simulink model "model_TugDynamics"  (R2023a)
settings: Solver=FixedStepAuto  StartTime=0.0  StopTime=400  FixedStep=0.025  RelTol=1e-3
model mask{StartTug=StartTug, Towline=0, Point=0}
  mask prompts: StartTug "Starting position [x y psi u v r]':"; Towline "Towline length:"; Point "Towline connection point Tanker [x_b y_b]':"
model workspace (MAT data in the model file):
  Point = [0; 0]
  Sig = Simulink.Signal
  Sig.DataType = 'auto'
  Sig.Dimensions = -1
  Sig.DimensionsMode = 'auto'
  Sig.Complexity = 'auto'
  Sig.SampleTime = -1
  Sig.SamplingMode = 'auto'
  StartTug = [0; 0; 0; 0; 0; 0]
  Towline = 0
  angleP = 0
  angleS = 0
  rpmP = 0
  rpmS = 0
undefined symbols (not defined in the file): TugStart
libraries: simulink x2
settings Model: ParameterArgumentNames=Point,StartTug,Towline  Creator=henni  LastModifiedBy=rkr021
settings OptimizationCC: ReuseModelBlockBuffer=off
settings DebuggingCC: UnconnectedInputMsg=warning  UnconnectedOutputMsg=warning  UnconnectedLineMsg=warning
settings ModelReferenceCC: EnableRefExpFcnMdlSchedulingChecks=on
settings RTWCC: DLArmComputeVersion=19.05

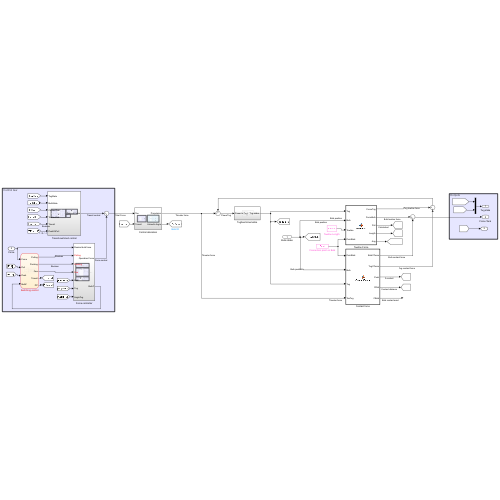
[thumbnail: Simulink's stored preview of the top-level diagram]
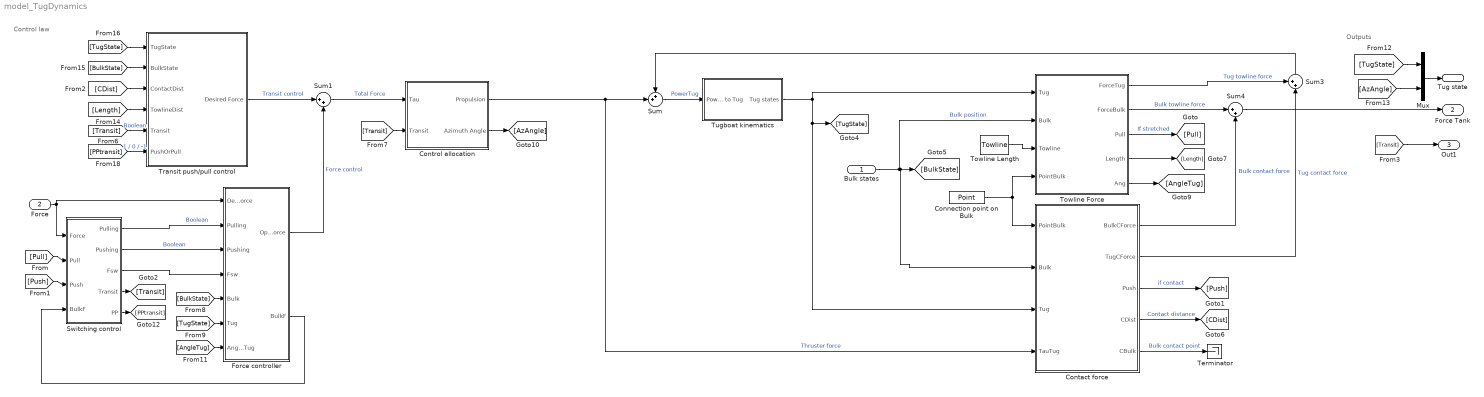
== system model_TugDynamics ==
  note: Outputs
  note: Control law
  Bulk states : Inport  PortDimensions=6
  Force : Inport  Port=2
  Connection point on Bulk : Constant  Value=Point
  Contact force : MATLAB Function  TreatAsAtomicUnit=on
  Control allocation : Subsystem
  Force controller : Subsystem
  Mux : Mux  Inputs=2
  Sum : Sum  Inputs=++|
  Sum1 : Sum  Inputs=|++
  Sum3 : Sum  Inputs=++|
  Sum4 : Sum  Inputs=|++
  Switching control : Stateflow chart  TreatAsAtomicUnit=on
  Terminator : Terminator
  Towline Force : MATLAB Function  TreatAsAtomicUnit=on
  Towline Length : Constant  Value=Towline
  Transit push/pull control : Subsystem
  Tugboat kinematics : Subsystem
  Tug state : Outport
  Force Tank : Outport  Port=2
  Out1 : Outport  Port=3
  wires:
  Sum3/1 -> Sum/1
  Tugboat kinematics/1(Tug states) -> Contact force/3(Tug), [TugState], Towline Force/1(Tug)
  Bulk states/1 -> [BulkState], Contact force/2(Bulk), Towline Force/2(Bulk)  "Bulk position"
  Sum4/1 -> Force Tank/1
  Towline Force/2(ForceBulk) -> Sum4/1  "Bulk towline force"
  Towline Length/1 -> Towline Force/3(Towline)
  Connection point on Bulk/1 -> Towline Force/4(PointBulk), Contact force/1(PointBulk)
  Contact force/1(BulkCForce) -> Sum4/2  "Bulk contact force"
  Towline Force/1(ForceTug) -> Sum3/1  "Tug towline force"
  Contact force/2(TugCForce) -> Sum3/2  "Tug contact force"
  Contact force/3(Push) -> [Push]  "if contact"
  Towline Force/3(Pull) -> [Pull]  "If stretched"
  Sum/1 -> Tugboat kinematics/1(Power to Tug)  "PowerTug"
  Control allocation/2(Azimuth Angle) -> [AzAngle]
  Control allocation/1(Propulsion) -> Contact force/4(TauTug), Sum/2  "Thruster force"
  Contact force/4(CDist) -> [CDist]  "Contact distance"
  Towline Force/4(Length) -> [Length]
  Contact force/5(CBulk) -> Terminator/1  "Bulk contact point"
  [Transit] -> Control allocation/2(Transit)
  Towline Force/5(Ang) -> [AngleTug]
  [TugState] -> Mux/1
  [AzAngle] -> Mux/2
  Mux/1 -> Tug state/1
  Switching control/3(Fsw) -> Force controller/4(Fsw)
  [PPtransit] -> Transit push/pull control/6(PushOrPull)  "1 / 0 / -1"
  [AngleTug] -> Force controller/7(AngleTug)
  [Push] -> Switching control/3(Push)
  [TugState] -> Force controller/6(Tug)
  Force/1 -> Switching control/1(Force), Force controller/1(Desired bulk force)
  Force controller/2(BulkF) -> Switching control/4(BulkF)
  Transit push/pull control/1(Desired Force) -> Sum1/1  "Transit control"
  [CDist] -> Transit push/pull control/3(ContactDist)
  [Transit] -> Transit push/pull control/5(Transit)  "Boolean"
  Switching control/2(Pushing) -> Force controller/3(Pushing)  "Boolean"
  [BulkState] -> Force controller/5(Bulk)
  Force controller/1(Operation Force) -> Sum1/2  "Force control"
  [Pull] -> Switching control/2(Pull)
  Switching control/5(PP) -> [PPtransit]
  Sum1/1 -> Control allocation/1(Tau)  "Total Force"
  Switching control/1(Pulling) -> Force controller/2(Pulling)  "Boolean"
  [Length] -> Transit push/pull control/4(TowlineDist)
  [TugState] -> Transit push/pull control/1(TugState)
  [BulkState] -> Transit push/pull control/2(BulkState)
  Switching control/4(Transit) -> [Transit]
  [Transit] -> Out1/1

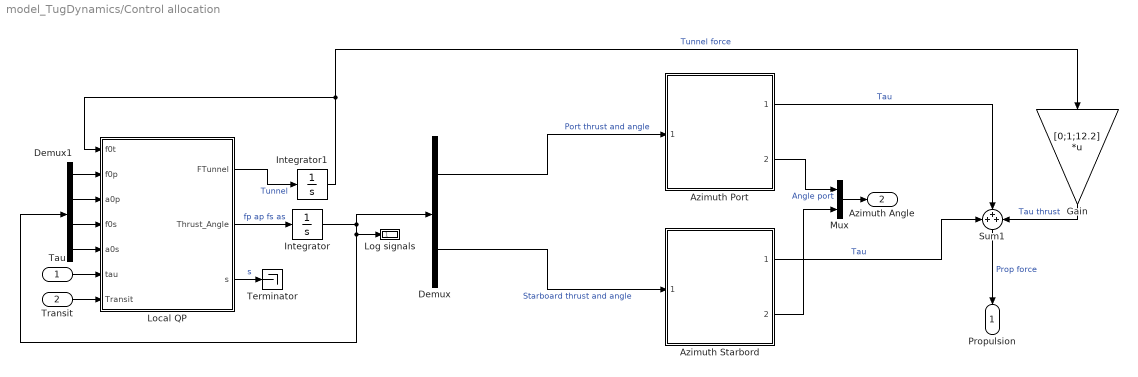
== system model_TugDynamics/Control allocation ==
  Tau : Inport  PortDimensions=3
  Transit : Inport  Port=2
  Azimuth Port : Subsystem  TreatAsAtomicUnit=on  ReferencedSubsystem=Subsystem_TugAzimuth  PosAz=[-13.9;-3]
  Azimuth Starbord : Subsystem  TreatAsAtomicUnit=on  ReferencedSubsystem=Subsystem_TugAzimuth  PosAz=[-13.9;3]
  Demux : Demux  Outputs=2
  Demux1 : Demux
  Gain : Gain  Gain=[0;1;12.2]  Multiplication=Matrix(K*u)
  Integrator : Integrator  InitialCondition=[0;deg2rad(0);0;deg2rad(-0)]
  Integrator1 : Integrator
  Local QP : MATLAB Function  TreatAsAtomicUnit=on
  Log signals : Subsystem
  Mux : Mux  Inputs=2
  Sum1 : Sum  Inputs=+++
  Terminator : Terminator
  Propulsion : Outport  PortDimensions=3
  Azimuth Angle : Outport  Port=2
  wires:
  Azimuth Port/1 -> Sum1/2  "Tau"
  Azimuth Starbord/1 -> Sum1/1  "Tau"
  Mux/1 -> Azimuth Angle/1
  Sum1/1 -> Propulsion/1  "Prop force"
  Demux/1 -> Azimuth Port/1  "Port thrust and angle"
  Integrator1/1 -> Gain/1, Local QP/1(f0t)  "Tunnel force"
  Integrator/1 -> Demux1/1, Log signals/1(Input), Demux/1
  Demux1/2 -> Local QP/3(a0p)
  Demux1/1 -> Local QP/2(f0p)
  Demux1/4 -> Local QP/5(a0s)
  Local QP/2(Thrust_Angle) -> Integrator/1  "fp ap fs as"
  Tau/1 -> Local QP/6(tau)
  Demux1/3 -> Local QP/4(f0s)
  Local QP/1(FTunnel) -> Integrator1/1  "Tunnel"
  Demux/2 -> Azimuth Starbord/1  "Starboard thrust and angle"
  Azimuth Port/2 -> Mux/1  "Angle port"
  Azimuth Starbord/2 -> Mux/2
  Transit/1 -> Local QP/7(Transit)
  Gain/1 -> Sum1/3  "Tau thrust"
  Local QP/3(s) -> Terminator/1  "s"

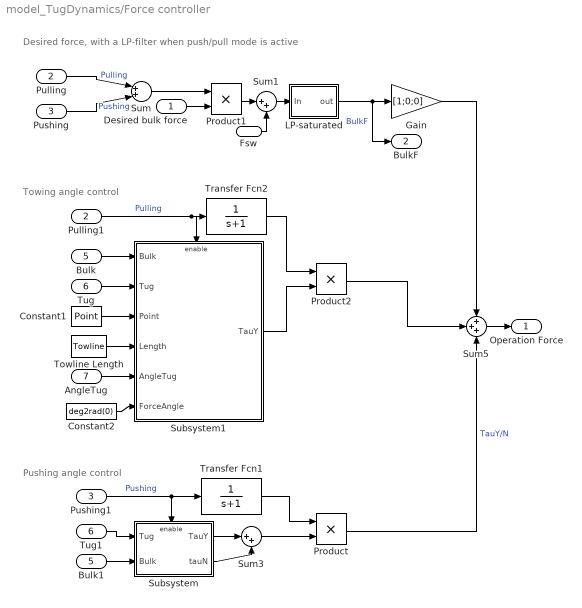
== system model_TugDynamics/Force controller ==
  note: Towing angle control
  note: Desired force, with a LP-filter when push/pull mode is active
  note: Pushing angle control
  Desired bulk force : Inport
  Pulling : Inport  Port=2
  Pushing : Inport  Port=3
  Fsw : Inport  Port=4
  Bulk : Inport  Port=5
  Tug : Inport  Port=6
  AngleTug : Inport  Port=7
  Bulk1 : InportShadow  Port=5
  Constant1 : Constant  Value=Point
  Constant2 : Constant  Value=deg2rad(0)
  Gain : Gain  Gain=[1;0;0]
  LP-saturated : Subsystem
  Product : Product
  Product1 : Product
  Product2 : Product
  Pulling1 : InportShadow  Port=2
  Pushing1 : InportShadow  Port=3
  Subsystem : Subsystem
  Subsystem1 : Subsystem
  Sum : Sum  Inputs=|++|
  Sum1 : Sum  Inputs=|++
  Sum3 : Sum  Inputs=|++
  Sum5 : Sum  Inputs=+++
  Towline Length : Constant  Value=Towline
  Transfer Fcn1 : TransferFcn  Denominator=[1 1]
  Transfer Fcn2 : TransferFcn  Denominator=[1 1]
  Tug1 : InportShadow  Port=6
  Operation Force : Outport
  BulkF : Outport  Port=2
  wires:
  Bulk1/1 -> Subsystem/2(Bulk)
  Pulling1/1 -> Subsystem1/Enable, Transfer Fcn2/1  "Pulling"
  Tug1/1 -> Subsystem/1(Tug)
  Constant1/1 -> Subsystem1/3(Point)
  Desired bulk force/1 -> Product1/2
  Transfer Fcn2/1 -> Product2/1
  Sum5/1 -> Operation Force/1
  Gain/1 -> Sum5/1
  Transfer Fcn1/1 -> Product/1
  Pulling/1 -> Sum/1  "Pulling"
  AngleTug/1 -> Subsystem1/5(AngleTug)
  Pushing/1 -> Sum/2  "Pushing"
  Bulk/1 -> Subsystem1/1(Bulk)
  Towline Length/1 -> Subsystem1/4(Length)
  Tug/1 -> Subsystem1/2(Tug)
  Product2/1 -> Sum5/2
  Product1/1 -> Sum1/1
  Fsw/1 -> Sum1/2
  LP-saturated/1(out) -> Gain/1, BulkF/1  "BulkF"
  Sum1/1 -> LP-saturated/1(In)
  Product/1 -> Sum5/3  "TauY/N"
  Constant2/1 -> Subsystem1/6(ForceAngle)
  Pushing1/1 -> Transfer Fcn1/1, Subsystem/Enable  "Pushing"
  Sum/1 -> Product1/1
  Subsystem/2(tauN) -> Sum3/2
  Subsystem/1(TauY) -> Sum3/1
  Sum3/1 -> Product/2
  Subsystem1/1(TauY) -> Product2/2

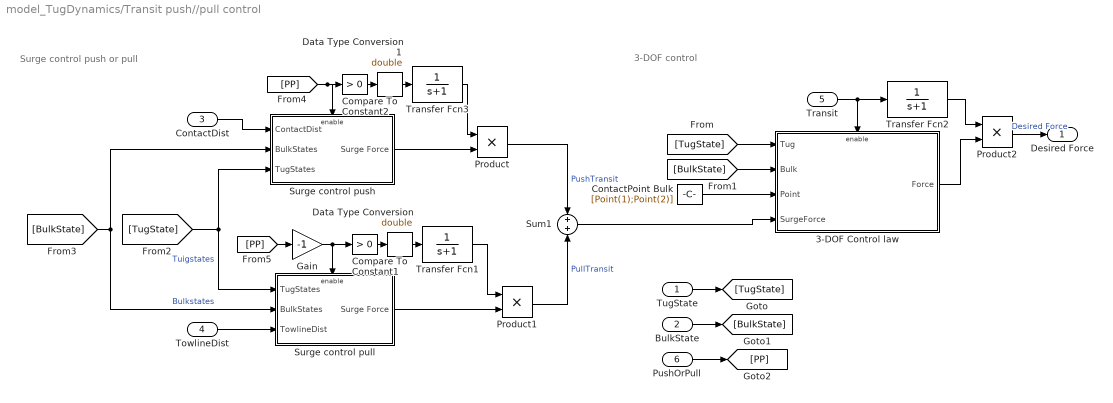
== system model_TugDynamics/Transit push//pull control ==
  note: 3-DOF control
  note: Surge control push or pull
  TugState : Inport
  BulkState : Inport  Port=2
  ContactDist : Inport  Port=3
  TowlineDist : Inport  Port=4
  Transit : Inport  Port=5
  PushOrPull : Inport  Port=6
  3-DOF Control law : Subsystem
  Compare To Constant1 : simulink/Logic and Bit Operations/Compare To Constant  relop=>  const=0  OutDataTypeStr=uint8
  Compare To Constant2 : simulink/Logic and Bit Operations/Compare To Constant  relop=>  const=0  OutDataTypeStr=uint8
  ContactPoint Bulk : Constant  Value=[Point(1);Point(2)]
  Data Type Conversion : DataTypeConversion  OutDataTypeStr=double  SaturateOnIntegerOverflow=off  RndMeth=Floor
  Data Type Conversion1 : DataTypeConversion  OutDataTypeStr=double  SaturateOnIntegerOverflow=off  RndMeth=Floor
  Gain : Gain  Gain=-1
  Product : Product
  Product1 : Product
  Product2 : Product
  Sum1 : Sum
  Surge control pull : Subsystem
  Surge control push : Subsystem
  Transfer Fcn1 : TransferFcn  Denominator=[1 1]
  Transfer Fcn2 : TransferFcn  Denominator=[1 1]
  Transfer Fcn3 : TransferFcn  Denominator=[1 1]
  Desired Force : Outport
  wires:
  [BulkState] -> Surge control pull/2(BulkStates), Surge control push/2(BulkStates)  "Bulkstates"
  Surge control pull/1(Surge Force) -> Product1/2
  [TugState] -> Surge control pull/1(TugStates), Surge control push/3(TugStates)  "Tuigstates"
  TowlineDist/1 -> Surge control pull/3(TowlineDist)
  ContactDist/1 -> Surge control push/1(ContactDist)
  TugState/1 -> [TugState]
  BulkState/1 -> [BulkState]
  PushOrPull/1 -> [PP]
  [PP] -> Compare To Constant2/1, Surge control push/Enable
  [PP] -> Gain/1
  Gain/1 -> Compare To Constant1/1, Surge control pull/Enable
  Surge control push/1(Surge Force) -> Product/2
  [TugState] -> 3-DOF Control law/1(Tug)
  [BulkState] -> 3-DOF Control law/2(Bulk)
  ContactPoint Bulk/1 -> 3-DOF Control law/3(Point)
  3-DOF Control law/1(" Force") -> Product2/2
  Transit/1 -> Transfer Fcn2/1, 3-DOF Control law/Enable
  Transfer Fcn3/1 -> Product/1
  Product/1 -> Sum1/1  "PushTransit"
  Compare To Constant1/1 -> Data Type Conversion/1
  Transfer Fcn1/1 -> Product1/1
  Product1/1 -> Sum1/2  "PullTransit"
  Transfer Fcn2/1 -> Product2/1
  Product2/1 -> Desired Force/1  "Desired Force"
  Sum1/1 -> 3-DOF Control law/4(SurgeForce)
  Data Type Conversion/1 -> Transfer Fcn1/1
  Data Type Conversion1/1 -> Transfer Fcn3/1
  Compare To Constant2/1 -> Data Type Conversion1/1

== system model_TugDynamics/Tugboat kinematics ==
  Power to Tug : Inport  PortDimensions=3
  Integrator : Integrator  InitialConditionSource=external  InitialCondition=[0;0;0;0;0;0]
  Kinematics CALC : MATLAB Function  TreatAsAtomicUnit=on
  initial state : Constant  Value=StartTug
  Tug states : Outport
  wires:
  Integrator/1 -> Kinematics CALC/1(x), Tug states/1  "x"
  Power to Tug/1 -> Kinematics CALC/2(tau)
  initial state/1 -> Integrator/2
  Kinematics CALC/1(xdot) -> Integrator/1  "xdot"

== system model_TugDynamics/Control allocation/Log signals ==
  Input : Inport
  Demux : Demux
  Gain1 : Gain  Gain=180/pi
  Gain2 : Gain  Gain=180/pi
  Mux1 : Mux
  Terminator : Terminator
  wires:
  Demux/2 -> Gain2/1  "Port angle"
  Mux1/1 -> Terminator/1  "PT PA ST SA"
  Gain2/1 -> Mux1/2  "Port angle"
  Demux/4 -> Gain1/1  "star angle"
  Gain1/1 -> Mux1/4  "star angle"
  Demux/3 -> Mux1/3  "Star thrust desired"
  Demux/1 -> Mux1/1  "Port Thrust desired"
  Input/1 -> Demux/1

== system model_TugDynamics/Force controller/LP-saturated ==
  In : Inport
  Integrator : Integrator
  Saturation : Saturate  UpperLimit=5e4  LowerLimit=-5e4
  Sum2 : Sum  Inputs=|+-
  out : Outport
  wires:
  Integrator/1 -> out/1, Sum2/2  "ut"
  Sum2/1 -> Saturation/1
  Saturation/1 -> Integrator/1
  In/1 -> Sum2/1

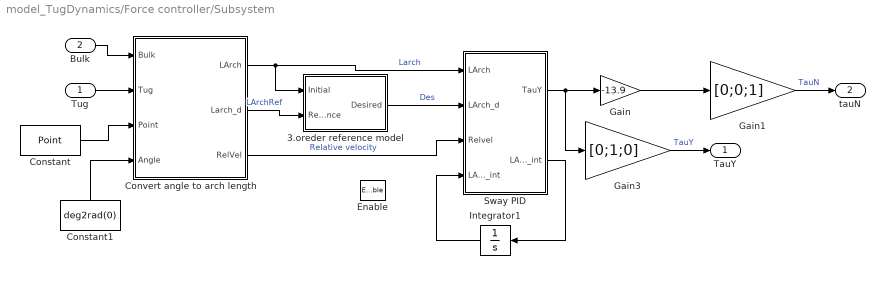
== system model_TugDynamics/Force controller/Subsystem ==
  Tug : Inport
  Bulk : Inport  Port=2
  Enable : EnablePort  StatesWhenEnabling=reset
  3.oreder reference model : Subsystem  mask{wn=0.02, zeta=1, sat_rd=0.4, sat_ad=0.01}
      mask prompts: wn "Natural frequency:"; zeta "Relative damping:"; sat_rd "Saturation eta_d_dot:"; sat_ad "Saturation eta_d_Ddot:"
  Constant : Constant  Value=Point
  Constant1 : Constant  Value=deg2rad(0)
  Convert angle to arch length : MATLAB Function  TreatAsAtomicUnit=on
  Gain : Gain  Gain=-13.9
  Gain1 : Gain  Gain=[0;0;1]
  Gain3 : Gain  Gain=[0;1;0]
  Integrator1 : Integrator
  Sway PID : MATLAB Function  TreatAsAtomicUnit=on
  TauY : Outport
  tauN : Outport  Port=2
  wires:
  Constant1/1 -> Convert angle to arch length/4(Angle)
  Gain1/1 -> tauN/1  "TauN"
  Gain3/1 -> TauY/1  "TauY"
  Tug/1 -> Convert angle to arch length/2(Tug)
  Constant/1 -> Convert angle to arch length/3(Point)
  Gain/1 -> Gain1/1
  Integrator1/1 -> Sway PID/4(LArch_int)
  Bulk/1 -> Convert angle to arch length/1(Bulk)
  Sway PID/2(LArch_error_int) -> Integrator1/1
  3.oreder reference model/1(Desired) -> Sway PID/2(LArch_d)  "Des"
  Convert angle to arch length/2(Larch_d) -> 3.oreder reference model/2(Reference)  "LArchRef"
  Convert angle to arch length/3(RelVel) -> Sway PID/3(Relvel)  "Relative velocity"
  Convert angle to arch length/1(LArch) -> 3.oreder reference model/1(Initial), Sway PID/1(LArch)  "Larch"
  Sway PID/1(TauY) -> Gain/1, Gain3/1

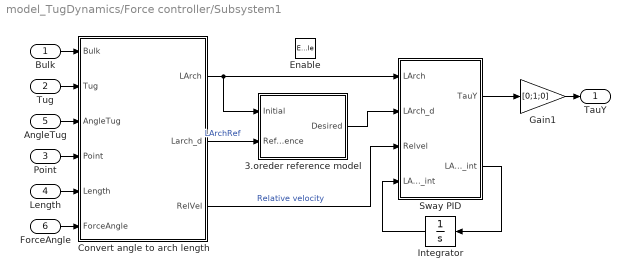
== system model_TugDynamics/Force controller/Subsystem1 ==
  Bulk : Inport
  Tug : Inport  Port=2
  Point : Inport  Port=3
  Length : Inport  Port=4
  AngleTug : Inport  Port=5
  ForceAngle : Inport  Port=6
  Enable : EnablePort  StatesWhenEnabling=reset
  3.oreder reference model : Subsystem  mask{wn=0.03, zeta=1, sat_rd=0.4, sat_ad=0.01}
      mask prompts: wn "Natural frequency:"; zeta "Relative damping:"; sat_rd "Saturation eta_d_dot:"; sat_ad "Saturation eta_d_Ddot:"
  Convert angle to arch length : MATLAB Function  TreatAsAtomicUnit=on
  Gain1 : Gain  Gain=[0;1;0]
  Integrator : Integrator
  Sway PID : MATLAB Function  TreatAsAtomicUnit=on
  TauY : Outport
  wires:
  Convert angle to arch length/1(LArch) -> Sway PID/1(LArch), 3.oreder reference model/1(Initial)
  Tug/1 -> Convert angle to arch length/2(Tug)
  ForceAngle/1 -> Convert angle to arch length/6(ForceAngle)
  Sway PID/1(TauY) -> Gain1/1
  Point/1 -> Convert angle to arch length/4(Point)
  Length/1 -> Convert angle to arch length/5(Length)
  Sway PID/2(LArch_error_int) -> Integrator/1
  Integrator/1 -> Sway PID/4(LArch_int)
  Bulk/1 -> Convert angle to arch length/1(Bulk)
  AngleTug/1 -> Convert angle to arch length/3(AngleTug)
  Convert angle to arch length/3(RelVel) -> Sway PID/3(Relvel)  "Relative velocity"
  Convert angle to arch length/2(Larch_d) -> 3.oreder reference model/2(Reference)  "LArchRef"
  3.oreder reference model/1(Desired) -> Sway PID/2(LArch_d)
  Gain1/1 -> TauY/1

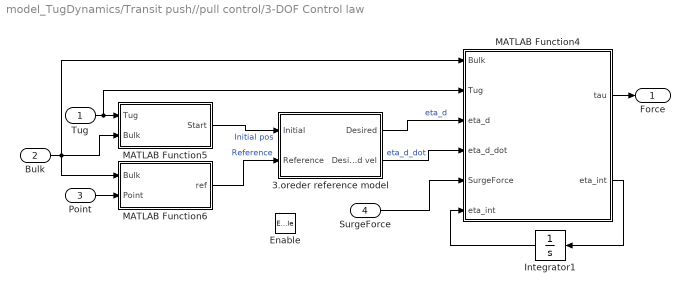
== system model_TugDynamics/Transit push//pull control/3-DOF Control law ==
  Tug : Inport
  Bulk : Inport  Port=2
  Point : Inport  Port=3
  SurgeForce : Inport  Port=4
  Enable : EnablePort  StatesWhenEnabling=reset
  3.oreder reference model : Subsystem  mask{wn=[0.1;0.1; 0.1], zeta=ones(3,1), sat_rd=[0.7;0.7;deg2rad(2)], sat_ad=[0.02;0.02;deg2rad(0.06)]}
      mask prompts: wn "Natural frequency:"; zeta "Relative damping:"; sat_rd "Saturation eta_d_dot:"; sat_ad "Saturation eta_d_Ddot:"
  Integrator1 : Integrator  InitialCondition=zeros(3,1)
  MATLAB Function4 : MATLAB Function  TreatAsAtomicUnit=on
  MATLAB Function5 : MATLAB Function  TreatAsAtomicUnit=on
  MATLAB Function6 : MATLAB Function  TreatAsAtomicUnit=on
  " Force" : Outport  PortDimensions=3
  wires:
  Integrator1/1 -> MATLAB Function4/6("eta_int ")
  Bulk/1 -> MATLAB Function4/1(Bulk), MATLAB Function5/2(Bulk), MATLAB Function6/1(Bulk)
  3.oreder reference model/1(Desired) -> MATLAB Function4/3(eta_d)  "eta_d"
  3.oreder reference model/2(Desired vel) -> MATLAB Function4/4(eta_d_dot)  "eta_d_dot"
  MATLAB Function5/1(Start) -> 3.oreder reference model/1(Initial)  "Initial pos"
  MATLAB Function6/1(ref) -> 3.oreder reference model/2(Reference)  "Reference"
  SurgeForce/1 -> MATLAB Function4/5(SurgeForce)
  Point/1 -> MATLAB Function6/2(Point)
  Tug/1 -> MATLAB Function4/2(Tug), MATLAB Function5/1(Tug)
  MATLAB Function4/2(eta_int) -> Integrator1/1
  MATLAB Function4/1(tau) -> " Force"/1

== system model_TugDynamics/Transit push//pull control/Surge control pull ==
  note: Surge velocity transit pull
  TugStates : Inport
  BulkStates : Inport  Port=2
  TowlineDist : Inport  Port=3
  Enable : EnablePort  StatesWhenEnabling=reset
  2.oreder reference model1 : Subsystem  mask{wn=0.15, zeta=1, sat_ad=0.04}
      mask prompts: wn "Natural frequency:"; zeta "Relative damping:"; sat_ad "Saturation v_d_dot:"
  ContactPoint : Constant  Value=[Point(1);Point(2)]
  Desired Velocity : MATLAB Function  TreatAsAtomicUnit=on
  Integrator5 : Integrator
  Towline : Constant  Value=Towline
  speedcontrol2 : MATLAB Function  TreatAsAtomicUnit=on
  Surge Force : Outport
  wires:
  Integrator5/1 -> speedcontrol2/5("e_int ")
  Desired Velocity/3(ud) -> 2.oreder reference model1/2(Reference)  "ref pull"
  TugStates/1 -> Desired Velocity/2(Tug)
  Desired Velocity/1(Int) -> speedcontrol2/1(Int)  "Check"
  Towline/1 -> Desired Velocity/5(Towline)
  BulkStates/1 -> Desired Velocity/1(Bulk)
  2.oreder reference model1/1(Desired) -> speedcontrol2/3(ud)  "Ud_pull"
  ContactPoint/1 -> Desired Velocity/3(Point)
  speedcontrol2/2(e_int) -> Integrator5/1
  TowlineDist/1 -> Desired Velocity/4(Length)
  speedcontrol2/1(ForceX) -> Surge Force/1
  2.oreder reference model1/2(Ud_dot) -> speedcontrol2/4(ud_dot)
  Desired Velocity/2(urel) -> 2.oreder reference model1/1(Initial), speedcontrol2/2(urel)  "urel pull"

== system model_TugDynamics/Transit push//pull control/Surge control push ==
  note: Surge velocity transit push
  ContactDist : Inport
  BulkStates : Inport  Port=2
  TugStates : Inport  Port=3
  Enable : EnablePort  StatesWhenEnabling=reset
  2.oreder reference model : Subsystem  mask{wn=0.15, zeta=1, sat_ad=0.04}
      mask prompts: wn "Natural frequency:"; zeta "Relative damping:"; sat_ad "Saturation v_d_dot:"
  ContactPoint : Constant  Value=[Point(1);Point(2)]
  Desired Velocity : MATLAB Function  TreatAsAtomicUnit=on
  Integrator1 : Integrator
  speedcontrol : MATLAB Function  TreatAsAtomicUnit=on
  Surge Force : Outport
  wires:
  speedcontrol/2(e_int) -> Integrator1/1
  BulkStates/1 -> Desired Velocity/1(Bulk)
  ContactPoint/1 -> Desired Velocity/3(Point)
  speedcontrol/1(ForceX) -> Surge Force/1
  ContactDist/1 -> Desired Velocity/4(CDist)
  Desired Velocity/3(ud) -> 2.oreder reference model/2(Reference)  "ref push"
  Integrator1/1 -> speedcontrol/5("e_int ")
  TugStates/1 -> Desired Velocity/2(Tug)
  2.oreder reference model/1(Desired) -> speedcontrol/3(ud)  "ud push"
  Desired Velocity/2(urel) -> 2.oreder reference model/1(Initial), speedcontrol/2(urel)  "urel push"
  Desired Velocity/1(Int) -> speedcontrol/1(Int)
  2.oreder reference model/2(Ud_dot) -> speedcontrol/4(ud_dot)

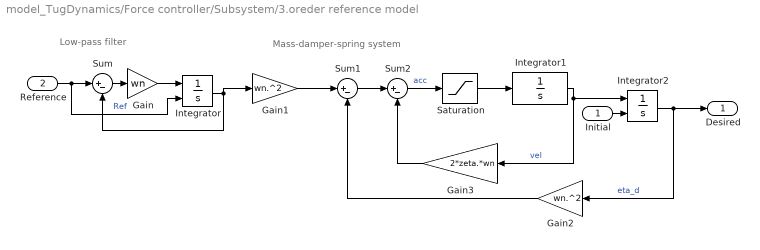
== system model_TugDynamics/Force controller/Subsystem/3.oreder reference model ==
  note: Mass-damper-spring system
  note: Low-pass filter
  Initial : Inport
  Reference : Inport  Port=2
  Gain : Gain  Gain=wn
  Gain1 : Gain  Gain=wn.^2
  Gain2 : Gain  Gain=wn.^2
  Gain3 : Gain  Gain=2*zeta.*wn
  Integrator : Integrator  InitialConditionSource=external  InitialCondition=TugStart
  Integrator1 : Integrator  LimitOutput=on  UpperSaturationLimit=sat_rd  LowerSaturationLimit=-sat_rd
  Integrator2 : Integrator  InitialConditionSource=external  InitialCondition=TugStart
  Saturation : Saturate  UpperLimit=sat_ad  LowerLimit=-sat_ad
  Sum : Sum  Inputs=|+-
  Sum1 : Sum  Inputs=|+-
  Sum2 : Sum  Inputs=|+-
  Desired : Outport
  wires:
  Sum1/1 -> Sum2/1
  Sum2/1 -> Saturation/1  "acc"
  Integrator1/1 -> Integrator2/1, Gain3/1  "vel"
  Integrator2/1 -> Desired/1, Gain2/1  "eta_d"
  Gain2/1 -> Sum1/2
  Gain3/1 -> Sum2/2
  Initial/1 -> Integrator2/2
  Saturation/1 -> Integrator1/1
  Reference/1 -> Integrator/2, Sum/1  "Ref"
  Integrator/1 -> Sum/2, Gain1/1
  Gain/1 -> Integrator/1
  Sum/1 -> Gain/1
  Gain1/1 -> Sum1/1

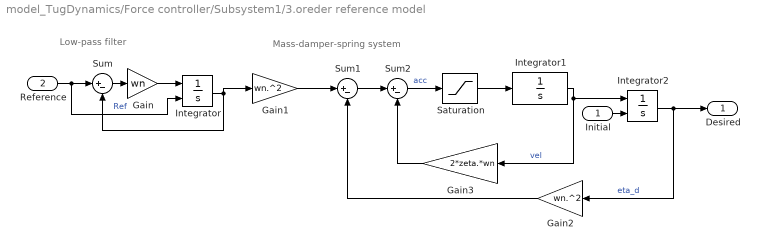
== system model_TugDynamics/Force controller/Subsystem1/3.oreder reference model ==
  note: Mass-damper-spring system
  note: Low-pass filter
  Initial : Inport
  Reference : Inport  Port=2
  Gain : Gain  Gain=wn
  Gain1 : Gain  Gain=wn.^2
  Gain2 : Gain  Gain=wn.^2
  Gain3 : Gain  Gain=2*zeta.*wn
  Integrator : Integrator  InitialConditionSource=external  InitialCondition=TugStart
  Integrator1 : Integrator  LimitOutput=on  UpperSaturationLimit=sat_rd  LowerSaturationLimit=-sat_rd
  Integrator2 : Integrator  InitialConditionSource=external  InitialCondition=TugStart
  Saturation : Saturate  UpperLimit=sat_ad  LowerLimit=-sat_ad
  Sum : Sum  Inputs=|+-
  Sum1 : Sum  Inputs=|+-
  Sum2 : Sum  Inputs=|+-
  Desired : Outport
  wires:
  Sum1/1 -> Sum2/1
  Sum2/1 -> Saturation/1  "acc"
  Integrator1/1 -> Integrator2/1, Gain3/1  "vel"
  Integrator2/1 -> Desired/1, Gain2/1  "eta_d"
  Gain2/1 -> Sum1/2
  Gain3/1 -> Sum2/2
  Initial/1 -> Integrator2/2
  Saturation/1 -> Integrator1/1
  Reference/1 -> Integrator/2, Sum/1  "Ref"
  Integrator/1 -> Sum/2, Gain1/1
  Gain/1 -> Integrator/1
  Sum/1 -> Gain/1
  Gain1/1 -> Sum1/1

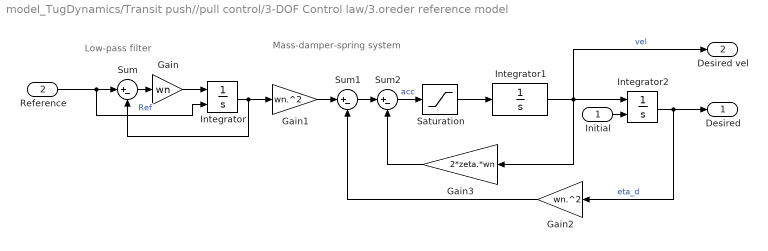
== system model_TugDynamics/Transit push//pull control/3-DOF Control law/3.oreder reference model ==
  note: Low-pass filter
  note: Mass-damper-spring system
  Initial : Inport
  Reference : Inport  Port=2
  Gain : Gain  Gain=wn
  Gain1 : Gain  Gain=wn.^2
  Gain2 : Gain  Gain=wn.^2
  Gain3 : Gain  Gain=2*zeta.*wn
  Integrator : Integrator  InitialConditionSource=external  InitialCondition=TugStart
  Integrator1 : Integrator  LimitOutput=on  UpperSaturationLimit=sat_rd  LowerSaturationLimit=-sat_rd
  Integrator2 : Integrator  InitialConditionSource=external  InitialCondition=TugStart
  Saturation : Saturate  UpperLimit=sat_ad  LowerLimit=-sat_ad
  Sum : Sum  Inputs=|+-
  Sum1 : Sum  Inputs=|+-
  Sum2 : Sum  Inputs=|+-
  Desired : Outport
  Desired vel : Outport  Port=2
  wires:
  Gain/1 -> Integrator/1
  Integrator/1 -> Gain1/1, Sum/2
  Sum/1 -> Gain/1
  Gain1/1 -> Sum1/1
  Sum1/1 -> Sum2/1
  Sum2/1 -> Saturation/1  "acc"
  Integrator1/1 -> Desired vel/1, Integrator2/1, Gain3/1  "vel"
  Integrator2/1 -> Desired/1, Gain2/1  "eta_d"
  Gain2/1 -> Sum1/2
  Gain3/1 -> Sum2/2
  Initial/1 -> Integrator2/2
  Saturation/1 -> Integrator1/1
  Reference/1 -> Integrator/2, Sum/1  "Ref"

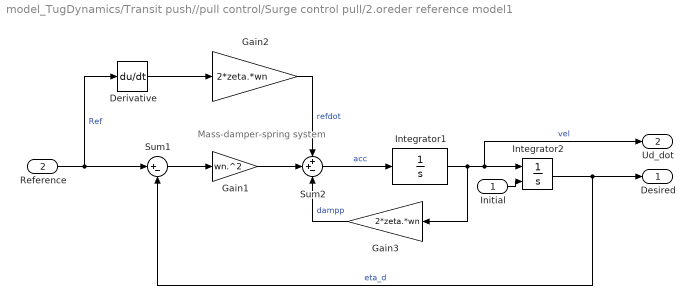
== system model_TugDynamics/Transit push//pull control/Surge control pull/2.oreder reference model1 ==
  note: Mass-damper-spring system
  Initial : Inport
  Reference : Inport  Port=2
  Derivative : Derivative
  Gain1 : Gain  Gain=wn.^2
  Gain2 : Gain  Gain=2*zeta.*wn
  Gain3 : Gain  Gain=2*zeta.*wn
  Integrator1 : Integrator  LimitOutput=on  UpperSaturationLimit=sat_ad  LowerSaturationLimit=-sat_ad
  Integrator2 : Integrator  InitialConditionSource=external  InitialCondition=TugStart
  Sum1 : Sum  Inputs=|+-
  Sum2 : Sum  Inputs=++-
  Desired : Outport
  Ud_dot : Outport  Port=2
  wires:
  Sum2/1 -> Integrator1/1  "acc"
  Integrator1/1 -> Gain3/1, Ud_dot/1, Integrator2/1  "vel"
  Integrator2/1 -> Sum1/2, Desired/1  "eta_d"
  Initial/1 -> Integrator2/2
  Gain1/1 -> Sum2/2
  Sum1/1 -> Gain1/1
  Reference/1 -> Derivative/1, Sum1/1  "Ref"
  Gain3/1 -> Sum2/3  "dampp"
  Derivative/1 -> Gain2/1
  Gain2/1 -> Sum2/1  "refdot"

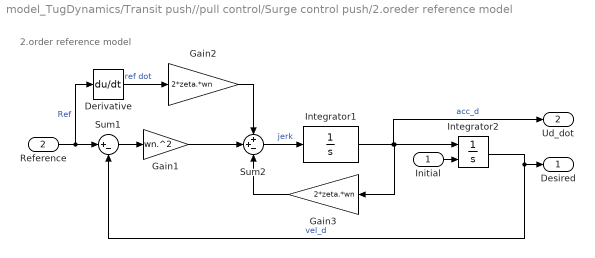
== system model_TugDynamics/Transit push//pull control/Surge control push/2.oreder reference model ==
  note: 2.order reference model
  Initial : Inport
  Reference : Inport  Port=2
  Derivative : Derivative
  Gain1 : Gain  Gain=wn.^2
  Gain2 : Gain  Gain=2*zeta.*wn
  Gain3 : Gain  Gain=2*zeta.*wn
  Integrator1 : Integrator  LimitOutput=on  UpperSaturationLimit=sat_ad  LowerSaturationLimit=-sat_ad
  Integrator2 : Integrator  InitialConditionSource=external  InitialCondition=TugStart
  Sum1 : Sum  Inputs=|+-
  Sum2 : Sum  Inputs=++-
  Desired : Outport
  Ud_dot : Outport  Port=2
  wires:
  Sum2/1 -> Integrator1/1  "jerk"
  Integrator1/1 -> Integrator2/1, Gain3/1, Ud_dot/1  "acc_d"
  Integrator2/1 -> Desired/1, Sum1/2  "vel_d"
  Initial/1 -> Integrator2/2
  Gain1/1 -> Sum2/2
  Sum1/1 -> Gain1/1
  Reference/1 -> Derivative/1, Sum1/1  "Ref"
  Gain3/1 -> Sum2/3
  Derivative/1 -> Gain2/1  "ref dot"
  Gain2/1 -> Sum2/1

== matlab function model_TugDynamics/Force controller/Subsystem/Convert angle to arch length ==
  data: Bulk input; Tug input; LArch output; Larch_d output; Point input; RelVel output; Angle input
function [LArch,Larch_d,RelVel] = fcn(Bulk,Tug,Point,Angle)


alpha = Tug(3)-Bulk(3);
                                                
alpha_d  = -sign(Point(2))*pi/2+Angle;                                  % Desired angle of attack, 90 deg out from the hull when there is no force angle

RelVel = -17.5*Tug(6);
LArch   = alpha*(17.5); 
Larch_d = alpha_d*(17.5);

== matlab function model_TugDynamics/Contact force ==
  data: PointBulk input; Bulk input; Tug input; BulkCForce output; TugCForce output; TauTug input; Push output; CDist output; CBulk output
function [BulkCForce, TugCForce, Push,CDist,CBulk] = ContactForce(PointBulk, Bulk, Tug, TauTug)
% -----Rotation matrices from body to NED -----% 
RBulk   = [cos(Bulk(3)), -sin(Bulk(3)); sin(Bulk(3)), cos(Bulk(3))];  
RTug    = [cos(Tug(3)), -sin(Tug(3)); sin(Tug(3)), cos(Tug(3))];
%  k_MFender = 7.438e7;


vec         = -sign(PointBulk(2))*RTug'*RBulk(:,2);         % Bulk body east vector represented in Tug body
CTug        = [11.75;0]+5.75*vec;                           % Position on TUG that will be in contact
CBulk1       = RBulk'*(Tug(1:2)+RTug*CTug-Bulk(1:2));       % Position of Bulk that will be in contact (x coordinate)
CBulk       = [CBulk1(1);PointBulk(2)];                     % Position in bulk body [xb; Chosen contact point]
CTug1       = RBulk'*(Tug(1:2)+RTug*CTug-Bulk(1:2));        % Tug contact point in bulk body
CDist       = -sign(PointBulk(2))*(CBulk(2)-CTug1(2));      % Impact distance, -sign(.) used to work on both sides of the bulk. 


frontback   = abs(CBulk(1))-123;                            % Ensures that the tugoat can drive in front or back of the vessel. 
if CDist <0 &&  frontback<0


    VBulk       = Bulk(4:5)+[-CBulk(2);CBulk(1)]*Bulk(6);                   % Velocity contact point Bulk
    VTug        =  Tug(4:5)+[-CTug(2);CTug(1)]*Tug(6);                      % Velocity contact point Tug
    vRsway     = sign(PointBulk(2))*(VBulk(2)-[0,1]*RBulk'*RTug*VTug);      % Relative velocity between tug and Bulk in sway (contact velocity)
    vRsurge      = VBulk(1)-[1,0]*RBulk'*RTug*VTug;                         % Relative velocity between tug and Bulk in surge (firction in sliding mode)
    velD = [RTug.'*RBulk*[VBulk(1);0];0];                                   % Velocity of the contacting point on bulk in surge direction, represented in Tugboat Body, assumed no rotation 
    dt=0.1;                                                                 % dt of 0.25 makes it oscilate in and out of the friction limit, 0.1 give similar results. 
    velD_dot = [RTug.'*RBulk*[vRsurge/dt;0];0];                             % Acceleration of points, as difference in velocity of contacting points in tugboa Body, assumed no rotation

    TugForce    = RBulk'*RTug*TauTug(1:2);                                  % Force from tug propulsion system on bulk carrier
    [M,C,D,Dn]=ContactFriction(velD);                                       % Finding the parameters for the tug contacting point to have the same velocity as contact point bulk
    stickForce = M*velD_dot+(C+D)*velD+Dn;                                  % Finding the required force for the tug
    stickDir = RBulk.'*RTug*stickForce(1:2);                                % Direction of forces represented in Bulk body
    VelDFric= (stickForce(1)^2+stickForce(2)^2)^(0.5)*sign(stickDir(1));    % This is not valid at side contact at port or stabord side, due to sign(0)



    %Curve fitting for the M-fender stiffness and resulting displacement
    %force. 
    A =abs(CDist)-[0; 0.05; 0.08; 0.095];       % Points on the curve, adding more stiffness
    C=A>0;                                      % Checking if the points has been crossed
    Steps = [4500e3;2167e3;5000e3;8333e3];      % Stiffness from curve fitting
    StiffForce=sum(A.*C.*Steps);                     % Curvefitted stiffness   
    Stiff = StiffForce/abs(CDist);
    
    CForce      = (StiffForce+0.1*sqrt(4*7.9e5*Stiff)*vRsway); % Contact force (Normal force)
    if CForce<0
        CForce=0;
    end

    CForce=-sign(PointBulk(2))*CForce;
    CFric       = (exp(-7*abs(vRsurge))*0.2+0.4)*abs(CForce);                       % Friction force, vR is the velocity of the sliding motion
    MaxFriction =   VelDFric-TugForce(1);   
    if abs(MaxFriction)<=CFric
        CFric       = MaxFriction;
        BulkForce   = -CFric;
    else
        CFric       = CFric*sign(MaxFriction);
        BulkForce   = -CFric;
    end
    
    FricTug     = [1,0;0,1,;-CTug(2),CTug(1)]*(RTug'*RBulk(:,1)*CFric);
    BulkCForce  = [1,0;0,1;-CBulk(2),CBulk(1)]*[BulkForce;CForce];
    TugCForce1  = [1,0;0,1;-CTug(2),CTug(1)]*(-vec*abs(CForce));
    TugCForce   = TugCForce1+FricTug;
    Push        = true;

else
    BulkCForce  = zeros(3,1);
    TugCForce   = zeros(3,1);
    Push        = false;
end


% k_MFender = 7.438e7

== matlab function model_TugDynamics/Force controller/Subsystem/Sway PID ==
  data: LArch input; LArch_d input; TauY output; Relvel input; LArch_int input; LArch_error_int output
function [TauY,LArch_error_int] = fcn(LArch,LArch_d, Relvel,LArch_int)
wb = 0.064; 
zeta=1;

[Kp,Kd,Ki] = TUG_SwayPIDGains(wb,zeta);
Error = LArch_d-LArch;
TauY = -Kp*Error-Kd*(Relvel)-Ki*LArch_int;
LArch_error_int = Error;

== matlab function model_TugDynamics/Tugboat kinematics/Kinematics CALC ==
  data: x input; xdot output; tau input
function xdot = fcn(x,tau)
% x = [eta;nu] = [xn;yn;psi;u;v;r]; 

[M,C,D,Dn,etaDot] = TugDynamicsCALC(x);
nu= x(4:6);
% U=sqrt(nu(1)^2+nu(2)^2);
nuDot  =M\(tau-C*nu-D*nu-Dn);

xdot = [etaDot;nuDot];

== matlab function model_TugDynamics/Towline Force ==
  data: ForceTug output; Tug input; Bulk input; Towline input; PointBulk input; ForceBulk output; Pull output; Length output; Ang output
function [ForceTug,ForceBulk,Pull,Length,Ang]=TowForce(Tug, Bulk, Towline, PointBulk)
% -----Rotation matrices from body to NED -----% 
% stiffness of towline
k_E         = 6.63e7;                                                       % 2% elongation and %3.315e7 with 4% elongation;  
RBulk       = [cos(Bulk(3)), -sin(Bulk(3)); sin(Bulk(3)), cos(Bulk(3))];    % Rotation from Bulk to Ned
RTug        = [cos(Tug(3)), -sin(Tug(3)); sin(Tug(3)), cos(Tug(3))];        % Rotation from Tug to Ned   
PointTug    = [17.5;0];                                                     % Towline connection tug represented in Body            
PosBulk     = Bulk(1:2)+RBulk*PointBulk;                                    % Towline connection bulk represented in NED 
PosTug      = Tug(1:2)+RTug*PointTug;                                       % Towline connection tug represented in NED 

Length      = sqrt((PosTug-PosBulk)'*(PosTug-PosBulk));                     % Distance between connection points

Vec         = (PosTug-PosBulk);                                             % Vector from tug to bulk connection
Ang         = atan2(Vec(2),Vec(1));                                         % The angle in NED

if Length >= Towline
% Vector force from Bulk and Tug
    %-----------------------------------------------%
    % Calculating the relative velocity in the direction of the towline tension. 
    VBulk       = Bulk(4:5)+[-PointBulk(2);PointBulk(1)]*Bulk(6);       % Velocity contact point Bulk
    VTug        =  Tug(4:5)+[-PointTug(2);PointTug(1)]*Tug(6);          % Velocity contact point tug
    VelNed      = RTug*VTug-RBulk*VBulk;                                % Relaative velocity in NED
    velTowline  = cos(Ang)*VelNed(1)+sin(Ang)*VelNed(2);          % Relative evlocity for stretching the towline
    %---------------------------------------------------%
    Force       = (Length-Towline)/Towline*k_E+(0.01*sqrt(4*7.9e5*k_E)*velTowline); % F = kx+dv, force in towline
    if Force <0    % Eliminate unwanted effects from the dissipative term in Force (dv), cant be negative.
        Force   = 0;                
    end

    VecBulk     = RBulk'*(PosTug-PosBulk);                                                      % Direction of force on Bulk
    AngBulk     = atan2(VecBulk(2),VecBulk(1)); 
    ForceBulk   = [1, 0; 0, 1; -PointBulk(2), PointBulk(1)]*[cos(AngBulk);sin(AngBulk)]*Force;  % Extended "thrust" coefficient matrix*force direction
   
    VecTug      = RTug'*(PosBulk-PosTug);                                                       % Direction of force on Tug
    AngTug      = atan2(VecTug(2),VecTug(1));
    ForceTug    = [1, 0; 0, 1; -PointTug(2), PointTug(1)]*[cos(AngTug);sin(AngTug)]*Force;      % Extended "thrust" coefficient matrix*force direction  
    Pull        = true; 
else
    ForceBulk   = zeros(3,1);
    ForceTug    = zeros(3,1);
    Pull        = false;
end

== stateflow chart model_TugDynamics/Switching control ==
  state TransitPush
    en, du:
    Transit = 1;
    PP=1;
    Fsw=0;
  state PushMode
    en, du:
    Pushing=1;
    PP=0;
    ex:
    Transit=1;
  state Stationary
    entry, during:
    Transit=1;
    Pushing=0;
    Pulling=0;
    PP=0;
    Fsw = 0;
  state PushReduction
    en,du:
    Fsw = -1e3;
  state PullReduction
    en,du:
    Fsw = 1e3;
  state PullMode
    en, du:
    Pulling=1;
    PP=0;
    ex:
    Transit = 1;
  state TransitPull
    en, du:
    Transit = 1;
    PP= -1;
    Fsw = 0;
  PushMode -> Stationary [order 1] : [Force==0]
  (default) -> Stationary
  TransitPush -> PushMode [order 1] : [Push==true]{Transit = 0;}
  Stationary -> TransitPush [order 1] : [Force>0]
  PushMode -> TransitPush [order 3] : [duration(Push==false)>15 ]{Pushing=0;}
  TransitPush -> Stationary [order 3] : [Force==0]
  TransitPush -> PushReduction [order 2] : [Force<0]{PP=0;}
  PushMode -> PushReduction [order 2] : [Force<0]{Pushing=0;}
  (junction 93) -> TransitPush
  PushReduction -> (junction 91) : [duration(BulkF<0)>5]
  (junction 91) -> TransitPull
  PullReduction -> (junction 93) : [duration(BulkF>0)>5]
  PullMode -> PullReduction [order 1] : [Force>0]{Pulling=0;}
  TransitPull -> PullReduction [order 2] : [Force>0]{PP=0;}
  Stationary -> TransitPull [order 2] : [Force<0]
  TransitPull -> Stationary [order 3] : [Force==0]
  TransitPull -> PullMode [order 1] : [Pull==true]{Transit = 0;}
  PullMode -> Stationary [order 2] : [Force==0]
  PullMode -> TransitPull [order 3] : [duration(Pull==false)>15]{Pulling=0;}
  data: Pulling output; Pushing output; Fsw output; Transit output; Force input; Pull input; Push input; BulkF input; PP output

== matlab function model_TugDynamics/Control allocation/Local QP ==
  data: f0t input; FTunnel output; f0p input; a0p input; Thrust_Angle output; f0s input; a0s input; tau input; Transit input; s output
function [FTunnel,Thrust_Angle,s]    = QPSolver(f0t,f0p, a0p, f0s, a0s, tau, Transit)

f0 = [f0t;f0p;f0s];
a0 = [a0p;a0s];

lyp = -3; lxp = -13.9; lys = 3; lxs = -13.9;
Tunnel = [0;1;12.2]*Transit;
T =     [Tunnel,   [cos(a0p),cos(a0s); 
                    sin(a0p),sin(a0s);
                    (-lyp*cos(a0p)+lxp*sin(a0p)),(-lys*cos(a0s)+lxs*sin(a0s))]];

dT = [-sin(a0p)*f0p,-sin(a0s)*f0s; 
         cos(a0p)*f0p,cos(a0s)*f0s;
         (lyp*sin(a0p)+lxp*cos(a0p))*f0p,(lys*sin(a0s)+lxs*cos(a0s))*f0s];


fLim = [-27e3,27e3; 0.01,30e4; 0.01,30e4];
aLim = deg2rad([0,180; -180,0]);
fRate = [27e3/2; 25e4/10; 25e4/10];
aRate = deg2rad([18;18]);

[df,da,s] = TugAlloc_lbub(tau,T, dT,f0,a0,fLim,aLim,fRate,aRate); % Improved, and used lower bound and upper bound to reduce size of the matrices. 

FTunnel = df(1);%+f0t;
Fp=df(2);%+f0p;
Fs = df(3);%+f0s;
Ap=da(1);%+a0p;
As=da(2);%+a0s;

Thrust_Angle = [Fp;   Ap;   Fs;   As];

== matlab function model_TugDynamics/Force controller/Subsystem1/Sway PID ==
  data: LArch input; LArch_d input; TauY output; Relvel input; LArch_int input; LArch_error_int output
function [TauY,LArch_error_int] = fcn(LArch,LArch_d, Relvel,LArch_int)
wb = 0.1; 
zeta=1;

[Kp,Kd,Ki] = TUG_SwayPIDGains(wb,zeta);
Error = LArch_d-LArch;
TauY = -Kp*Error-Kd*(Relvel)-Ki*LArch_int;

LArch_error_int = Error;

== matlab function model_TugDynamics/Force controller/Subsystem1/Convert angle to arch length ==
  data: Bulk input; Tug input; LArch output; Larch_d output; AngleTug input; Point input; Length input; ForceAngle input; RelVel output
function [LArch,Larch_d,RelVel] = fcn(Bulk,Tug,AngleTug,Point,Length,ForceAngle)

alpha = AngleTug-Bulk(3);                                                   % Current angle of attack, towline angle from bulk
alpha_d  = sign(Point(2))*pi/2+ForceAngle;                          % Desired angle of attack, 90 deg out from the hull when there is no force angle

TowPBulk = Point+(Length+17.5)*[cos(alpha_d);sin(alpha_d)];                 % Towing point +17.5(CO) in bulk reference frame, used o find the velocity 
Ralpd = [cos(alpha_d),-sin(alpha_d); sin(alpha_d),cos(alpha_d)];            % Rotation matrix for the desired angle of attack, used to find velocity of point

TowPointVel = [0,1]*Ralpd'*(Bulk(4:5)+[-TowPBulk(2);TowPBulk(1)]*Bulk(6));  % Velocity in the direction of the curvature of the towline The ARCH, at distance Towline + Tuggboat CO (17.5)

Ralph = [cos(alpha),-sin(alpha); sin(alpha),cos(alpha)];  
RTug = [cos(Tug(3)),-sin(Tug(3)); sin(Tug(3)),cos(Tug(3))];  
RBulk = [cos(Bulk(3)),-sin(Bulk(3)); sin(Bulk(3)),cos(Bulk(3))];  

TugpointVel = [0,1]*Ralph'*RBulk'*RTug*(Tug(4:5));                          % Tugboat sway velocity converted to the current anlge of attack

RelVel = TowPointVel-TugpointVel;                                % Relative velocity that the tug closes inn on the desired angle of attack towing point.


LArch   = alpha*(Length+17.5); 
Larch_d = alpha_d*(Length+17.5);

== matlab function model_TugDynamics/Transit push//pull control/Surge control push/speedcontrol ==
  data: Int input; urel input; ForceX output; ud input; ud_dot input; e_int input; e_int output
function [ForceX,e_int] = fcn(Int, urel, ud,ud_dot, e_int)

wb = 0.19; zeta = 1;
[Msurge,Kp,Ki] = TUG_SurgePI(wb,zeta);
if Int==0
    ForceX =0;
    e_int = 0;
else
    e = ud-urel;
    ForceX = Kp*e+Ki*e_int+Msurge*ud_dot;
    e_int=e;
end

== matlab function model_TugDynamics/Transit push//pull control/Surge control push/Desired Velocity ==
  data: Int output; urel output; ud output; Bulk input; Tug input; Point input; CDist input
function [Int, urel, ud]   = fcn(Bulk,Tug,Point,CDist)
RBulk   = [cos(Bulk(3)), -sin(Bulk(3)); sin(Bulk(3)), cos(Bulk(3))];
RTug   = [cos(Tug(3)), -sin(Tug(3)); sin(Tug(3)), cos(Tug(3))];

Dist =  RBulk.'*(Tug(1:2)-Bulk(1:2));
Heading = ssa((Bulk(3)-sign(Point(2))*pi/2)-Tug(3));
xtilde = abs(Dist(1)-Point(1)); % Distance from surge coordinate, reached with 3DOF controller.
velPoint = Bulk(4:5)+[-Point(2);Point(1)]*Bulk(6);  % velocity between tug ang bulk
urel = sign(Point(2))*(velPoint(2)-[0,1]*RBulk'*RTug*Tug(4:5)); % relative velocity between tug ang bulk

if CDist<0
    CDist=0;
end

ud = urel+(1.2*(1-exp(-CDist/30))+0.1-urel)*exp(-xtilde/2)*exp(-abs(0.5*Heading*180/pi));
if xtilde<10
Int = 1;
else
    Int =0;
end

== matlab function model_TugDynamics/Transit push//pull control/3-DOF Control law/MATLAB Function4 ==
  data: Bulk input; Tug input; eta_d input; eta_d_dot input; SurgeForce input; tau output; eta_int input; eta_int output
function [tau,eta_int]    = DOF3Body(Bulk, Tug, eta_d,eta_d_dot, SurgeForce,eta_int)

eta = Tug(1:3);
nu  = Tug(4:6);
wb = [0.2;0.2;0.3];
zeta = ones(3,1);

[Kp,Kd,Ki] = TugPID_Gains(wb,zeta,eta(3)-Bulk(3),nu);

RTug    = [cos(Tug(3)), -sin(Tug(3)); sin(Tug(3)), cos(Tug(3))];
RBulk   = [cos(Bulk(3)), -sin(Bulk(3)); sin(Bulk(3)), cos(Bulk(3))];
Dist =  RBulk.'*(Tug(1:2)-Bulk(1:2));
eta_tilde = [Dist(1)-eta_d(1);0;eta(3)-eta_d(3)];

ye_dot = RBulk'*RTug*nu(1:2)-Bulk(4:5);



eta_tilde_dot =  [ye_dot(1);0;nu(3)]-eta_d_dot;
eta_tilde(3) = ssa(eta_tilde(3));
    RRTug =Rzyx(0,0,eta(3));
    RRBulk =Rzyx(0,0,Bulk(3));
    PIDtau = -Kp*eta_tilde-Kd*eta_tilde_dot-Ki*eta_int;
    eta_int =eta_tilde;

    tau=RRTug'*RRBulk*PIDtau+[SurgeForce;0;0];

== matlab function model_TugDynamics/Transit push//pull control/3-DOF Control law/MATLAB Function5 ==
  data: Tug input; Bulk input; Start output
function Start=InitialPos(Tug,Bulk)
RBulk   = [cos(Bulk(3)), -sin(Bulk(3)); sin(Bulk(3)), cos(Bulk(3))];

Pos = RBulk.'*(Tug(1:2)-Bulk(1:2));
Start= [Pos(1);0;Tug(3)];

== matlab function model_TugDynamics/Transit push//pull control/Surge control pull/Desired Velocity ==
  data: Int output; urel output; ud output; Bulk input; Tug input; Point input; Length input; Towline input
function [Int,urel, ud]   = fcn(Bulk,Tug,Point,Length, Towline)
RBulk   = [cos(Bulk(3)), -sin(Bulk(3)); sin(Bulk(3)), cos(Bulk(3))];
RTug   = [cos(Tug(3)), -sin(Tug(3)); sin(Tug(3)), cos(Tug(3))];

Dist =  RBulk.'*(Tug(1:2)-Bulk(1:2));
Heading = ssa((Bulk(3)-sign(Point(2))*pi/2)-Tug(3));
xtilde = abs(Dist(1)-Point(1)); % Distance from surge coordinate, reached with 3DOF controller.
velPoint = Bulk(4:5)+[-Point(2);Point(1)]*Bulk(6);  % velocity between tug ang bulk
% VelRel = RBulk.'*RTug*Tug(4:5)-velPoint;            % relative velocity between tug ang bulk
% urel = VelRel(2);                                   % velocity in bulk body surge direction
urel = sign(Point(2))*(velPoint(2)-[0,1]*RBulk'*RTug*Tug(4:5)); % relative velocity between tug ang bulk     
TDist = Towline-Length;

if TDist<0
    TDist=0;
end

ud = urel+(-1.2*(1-exp(-TDist/30))-0.1-urel)*exp(-xtilde/2)*exp(-abs(0.5*Heading*180/pi));
if xtilde<10
Int = 1;
else
    Int =0;
end

== matlab function model_TugDynamics/Transit push//pull control/3-DOF Control law/MATLAB Function6 ==
  data: Bulk input; ref output; Point input
function ref  = Reference(Bulk,Point)
% % 
% RBulk   = [cos(Bulk(3)), -sin(Bulk(3)); sin(Bulk(3)), cos(Bulk(3))];


pi_p=Bulk(3)-sign(Point(2))*pi/2;%atan2(pi_p(2),pi_p(1));
% Dist =  RBulk.'*(Tug(1:2)-Bulk(1:2));
% Ke = 0.0000002;
% pi_p=pi_p+atan(Ke*(Dist(1)^4)*sign(Dist(1)));
ref = [Point(1);0;pi_p];
% vel = Bulk(4:5)+[-Point(2);Point(1)]*Bulk(6);    
% ref_dot= [vel(1);0;Bulk(6)];

== matlab function model_TugDynamics/Transit push//pull control/Surge control pull/speedcontrol2 ==
  data: Int input; urel input; ForceX output; ud input; ud_dot input; e_int input; e_int output
function [ForceX,e_int] = fcn(Int,urel, ud,ud_dot, e_int)

wb = 0.19; zeta = 1;
[Msurge,Kp,Ki] = TUG_SurgePI(wb,zeta);
if Int==0
    ForceX =0;
    e_int = 0;
else
    e = ud-urel;
    ForceX = Kp*e+Ki*e_int+Msurge*ud_dot;
    e_int=e;
end
